simulink model "Sennels_mWave"  (R2014a)
settings: Solver=FixedStepDiscrete  StartTime=0.0  StopTime=10  FixedStep=1/3333  RelTol=1e-3
libraries: dspmtrx3 x2, dspinverses x1
settings Model: Creator=bethel.osuagwu  LastModifiedBy=bethel.osuagwu

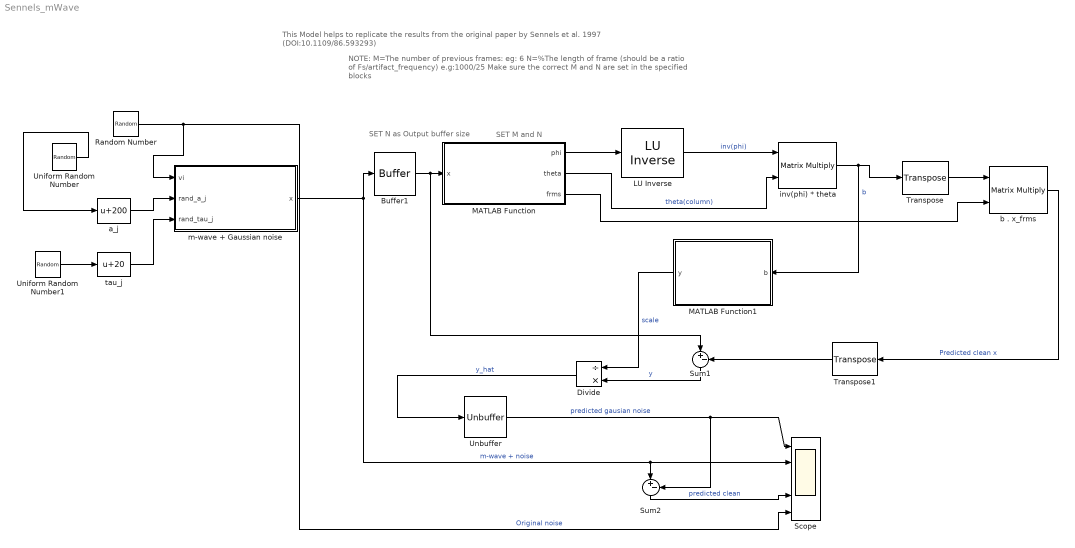
== system Sennels_mWave ==
  note: NOTE:
      | M=The number of previous frames: eg: 6
      | N=%The length of frame (should be a ratio of Fs/artifact_frequency) e.g:1000/25
      | Make sure the correct M and N are set in the specified blocks
  note: SET N as Output
      | buffer size
  note: SET M and N
  note: This Model helps to replicate the results from the original paper by Sennels et al. 1997 (DOI:10.1109/86.593293)
  " LU Inverse" : dspinverses/ LU Inverse
  Buffer1 : Buffer  N=111  TreatMby1Signals=One channel
  Divide : Product  Inputs=/*
  MATLAB Function : MATLAB Function  TreatAsAtomicUnit=on
  MATLAB Function1 : MATLAB Function  TreatAsAtomicUnit=on
  Random Number : RandomNumber  SampleTime=1/3333
  Scope : Scope  NumInputPorts=5
      settings: ShowLegends=on  YMin=-25~-75~-1~-75~-4  YMax=25~175~1~200~5
  Sum1 : Sum  Inputs=|+-
  Sum2 : Sum  Inputs=|+-
  Transpose : dspmtrx3/Transpose  Hermitian=off  overflowFlag=off
  Transpose1 : dspmtrx3/Transpose  Hermitian=off  overflowFlag=off
  Unbuffer : Unbuffer  SampleBasedProcessing=Same as frame based
  Uniform Random Number : UniformRandomNumber  Minimum=-200*0.5  Maximum=200*0.5  SampleTime=1/3333
  Uniform Random Number1 : UniformRandomNumber  Minimum=-20*0.4  Maximum=20*0.5  SampleTime=1/3333
  a_j : Bias  Bias=200
  b . x_frms : Product  Multiplication=Matrix(*)
  inv(phi) * theta : Product  Multiplication=Matrix(*)
  m-wave + Gaussian noise : MATLAB Function  TreatAsAtomicUnit=on
  tau_j : Bias  Bias=20
  wires:
  Buffer1/1 -> Sum1/1, MATLAB Function/1(x)
  MATLAB Function/1(phi) -> " LU Inverse"/1
  MATLAB Function/2(theta) -> inv(phi) * theta/2  "theta(column)"
  " LU Inverse"/1 -> inv(phi) * theta/1  "inv(phi)"
  inv(phi) * theta/1 -> MATLAB Function1/1(b), Transpose/1  "b"
  Unbuffer/1 -> Sum2/2, Scope/1  "predicted gausian noise"
  MATLAB Function/3(frms) -> b . x_frms/2
  Transpose/1 -> b . x_frms/1
  b . x_frms/1 -> Transpose1/1  "Predicted clean x"
  Random Number/1 -> m-wave + Gaussian noise/1(vi), Scope/5  "Original noise"
  m-wave + Gaussian noise/1(x) -> Sum2/1, Scope/2, Buffer1/1  "m-wave + noise"
  Uniform Random Number/1 -> a_j/1
  Uniform Random Number1/1 -> tau_j/1
  a_j/1 -> m-wave + Gaussian noise/2(rand_a_j)
  tau_j/1 -> m-wave + Gaussian noise/3(rand_tau_j)
  Transpose1/1 -> Sum1/2
  Sum1/1 -> Divide/2  "y"
  MATLAB Function1/1(y) -> Divide/1  "scale"
  Divide/1 -> Unbuffer/1  "y_hat"
  Sum2/1 -> Scope/4  "predicted clean"

== matlab function Sennels_mWave/MATLAB Function1 ==
  data: b input; y output
function y = fcn(b)
%#codegen


y = sqrt(1+sum(b.^2));
%       OR
%y = (1+sum(b));%approximated for speed

== matlab function Sennels_mWave/MATLAB Function ==
  data: x input; phi output double; theta output; frms output
function [phi,theta,frms] = fcn(x)
%#codegen
persistent t_sample phi_mem  frms_mem ;

%General param
M=6; %The number of previous frames 
N=111; %The length of frame (should be a ratio of Fs/artifact_frequency)

% Performance parameter
freshPhi =1;% when =1:recompute phi(covariance matix) all the phi; when =0:update phi with only new values

if isempty(t_sample)
    t_sample=0;
    frms_mem=zeros(M,N);
    
    phi_mem=zeros(M,M);
end
t_sample=t_sample+1;

%make x a row vector
x=x';


%% compute phi
frms=frms_mem;
%equ 7 and 8
if(freshPhi)
    % compute phi fresh all the time
    phi=(frms*frms');
else
    %we can compute only the required column (first) and row (first)of phi
    %matrix and push the new values into phi
    phi_mem(2:end,2:end)=phi_mem(1:end-1,1:end-1);
    phi_mem(1,:)=frms(1,:)*frms';
    phi_mem(:,1)=phi_mem(1,:)';
    %phi-phi_mem
    phi=phi_mem;
end


%% compute theta
theta=(x*frms')';
%t_sample
%if t_sample==15
%    y=4;
%end


%% update frame
frms_mem(2:end,:)=frms_mem(1:end-1,:);
frms_mem(1,:)=x;

== matlab function Sennels_mWave/m-wave + Gaussian noise ==
  data: x output; vi input; rand_a_j input; rand_tau_j input
function x = fcn(vi,rand_a_j,rand_tau_j)
%#codegen
persistent t i tau_j_mem a_j_mem;
N=111;
if isempty(t)
    t=0;
    i=0;
    
    a_j_mem=200;    
    tau_j_mem=20;
    
end
t=t+1;


i=i+1;
if i==N
    i=0;
    
    %there param are only changed at the begining of each frame
    tau_j_mem=rand_tau_j;
    a_j_mem=rand_a_j;
end

tau_j=tau_j_mem;
%tau_j=20;%open this to keep it constant
a_j=a_j_mem;
a_j=200;%open this to keep it constant


x=( a_j*exp(-i/tau_j)*sin(2*pi*3*i/N) )+vi;
